simulink model "V_1_FuzzyCode"  (R2025b)
settings: Solver=VariableStepAuto  StartTime=0.0  StopTime=10.0  RelTol=1e-3
settings Model: Creator=acer  LastModifiedBy=acer

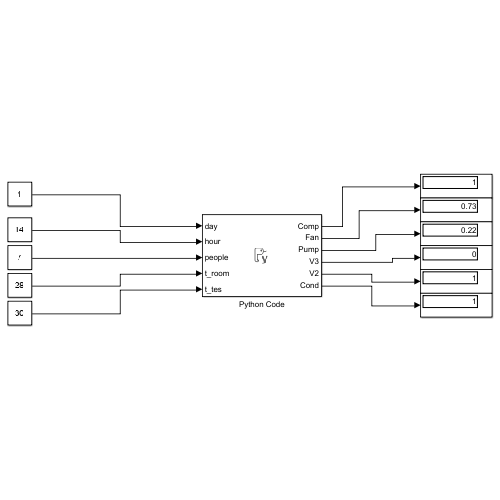
[thumbnail: Simulink's stored preview of the top-level diagram]
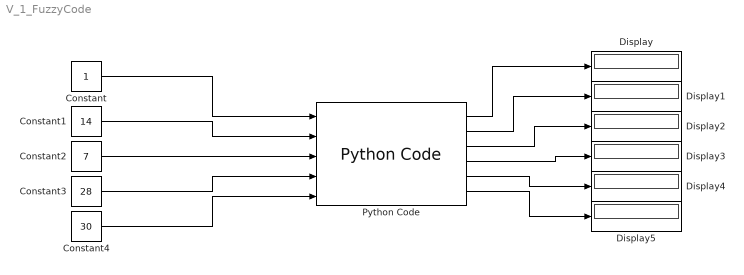
== system V_1_FuzzyCode ==
  Constant : Constant
  Constant1 : Constant  Value=14
  Constant2 : Constant  Value=7
  Constant3 : Constant  Value=28
  Constant4 : Constant  Value=30
  Display{,1..5} (6 alike) : Display
  Python Code : PythonCode  OutputCode=|
      | import numpy as np
      | import skfuzzy as fuzz
      | from skfuzzy import control as ctrl
      | 
      | # ==========================================================
      | # Persistent Fuzzy System (สร้างครั้งเดียว)
      | # ==========================================================
      | def create_fuzzy_system():
      | 
      |     # -------- INPUTS --------
      |     people = ctrl.Antecedent(np.arange(1, 32, 1), 'people')
      |     room_temp = ctrl.Antecedent(np.arange(20, 31, 1), 'room_temp')
      | 
      |     # -------- OUTPUTS --------
      |     cond_use = ctrl.Consequent(np.arange(0, 1.1, 0.1), 'cond_use')
      |     comp_use = ctrl.Consequent(np.arange(0, 1.1, 0.1), 'comp_use')
      |     pump_speed = ctrl.Consequent(np.arange(0, 101, 1), 'pump_speed')
      |     fan_speed = ctrl.Consequent(np.arange(0, 101, 1), 'fan_speed')
      |     valve_2 = ctrl.Consequent(np.arange(0, 1.1, 0.1), 'valve_2')
      |     valve_3 = ctrl.Consequent(np.arange(0, 1.1, 0.1), 'valve_3')
      | 
      |     # -------- MEMBERSHIP FUNCTIONS --------
      |     people['few'] = fuzz.trapmf(people.universe, [0, 0, 4, 6])
      |     people['medium'] = fuzz.trapmf(people.universe, [5, 10, 15, 15])
      |     people['many'] = fuzz.trapmf(people.universe, [14, 25, 31, 31])
      | 
      |     room_temp['normal'] = fuzz.trimf(room_temp.universe, [20, 20, 26])
      |     room_temp['hot'] = fuzz.trimf(room_temp.universe, [24, 27, 29])
      |     room_temp['very_hot'] = fuzz.trapmf(room_temp.universe, [28, 29, 30, 30])
      | 
      |     for output in [cond_use, comp_use, valve_2, valve_3]:
      |         output['off'] = fuzz.trimf(output.universe, [0, 0, 0.5])
      |         output['on']  = fuzz.trimf(output.universe, [0.5, 1, 1])
      | 
      |     pump_speed['low'] = fuzz.trimf(pump_speed.universe, [0, 30, 40])
      |     pump_speed['high'] = fuzz.trimf(pump_speed.universe, [30, 100, 100])
      | 
      |     fan_speed['low'] = fuzz.trimf(fan_speed.universe, [0, 30, 40])
      |     fan_speed['high'] = fuzz.trimf(fan_speed.universe, [30, 100, 100])
      | 
      |     # -------- RULES --------
      |     rules = [
      | 
      |         ctrl.Rule(people['few'] & room_temp['normal'],
      |                   [cond_use['off'], comp_use['off'], pump_speed['low'],
      |                    fan_speed['low'], valve_2['off'], valve_3['off']]),
      | 
      |         ctrl.Rule(people['medium'] & room_temp['hot'],
      |                   [cond_use['on'], comp_use['on'], pump_speed['low'],
      |                    fan_speed['high'], valve_2['on'], valve_3['off']]),
      | 
      |         ctrl.Rule(people['many'] & room_temp['very_hot'],
      |                   [cond_use['on'], comp_use['on'], pump_speed['high'],
      |                    fan_speed['high'], valve_2['on'], valve_3['off']])
      |     ]
      | 
      |     system = ctrl.ControlSystem(rules)
      |     return ctrl.ControlSystemSimulation(system)
      | 
      | 
      | # ==========================================================
      | # Controller (Time-Step Function)
      | # ==========================================================
      | fuzzy_sim = create_fuzzy_system()
      | 
      | def tes_controller(day, hour, people, t_room, t_tes):
      |     """
      |     Time-step controller (เรียกครั้งละ 1 timestep)
      | 
      |     Inputs:
      |         day     : 0-6
      |         hour    : 0-23
      |         people  : จำนวนคน
      |         t_room  : อุณหภูมิห้อง (°C)
      |         t_tes   : อุณหภูมิถัง (°C)
      | 
      |     Returns:
      |         cond, v2, v3, pump, fan, comp
      |     """
      | 
      |     # Default Output
      |     cond = 0
      |     v2 = 0
      |     v3 = 0
      |     pump = 0
      |     fan = 0
      |     comp = 0
      | 
      |     # ==============================
      |     # MODE 1 : Night Charging
      |     # ==============================
      |     if hour >= 22 or hour < 9:
      | 
      |         if people < 1:
      |             if t_tes > 5:
      |                 cond = 1
      |                 v3 = 1
      |                 comp = 1
      |         else:
      |             if t_tes > 5 and t_room > 24:
      |                 cond = 1
      |                 v2 = 1
      |                 v3 = 1
      |                 fan = 1
      |                 comp = 1
      |             elif t_tes > 5:
      |                 cond = 1
      |                 v3 = 1
      | 
      |     # ==============================
      |     # MODE 2 : Day Operation
      |     # ==============================
      |     else:
      | 
      |         if t_room > 24:
      | 
      |             fuzzy_sim.input['people'] = people
      |             fuzzy_sim.input['room_temp'] = t_room
      |             fuzzy_sim.compute()
      | 
      |             cond = int(fuzzy_sim.output['cond_use'] >= 0.5)
      |             comp = int(fuzzy_sim.output['comp_use'] >= 0.5)
      |             v2   = int(fuzzy_sim.output['valve_2'] >= 0.5)
      |             v3   = int(fuzzy_sim.output['valve_3'] >= 0.5)
      | 
      |             pump = round(fuzzy_sim.output['pump_speed'] / 100, 2)
      |             fan  = round(fuzzy_sim.output['fan_speed'] / 100, 2)
      | 
      |     return cond, v2, v3, pump, fan, comp
      | 
      | Cond,V2,V3,Pump,Fan,Comp = tes_controller(1, 14, 12, 28, 7)
  wires:
  Python Code/1 -> Display/1
  Constant/1 -> Python Code/1
  Constant1/1 -> Python Code/2
  Constant3/1 -> Python Code/4
  Constant2/1 -> Python Code/3
  Constant4/1 -> Python Code/5
  Python Code/2 -> Display1/1
  Python Code/3 -> Display2/1
  Python Code/4 -> Display3/1
  Python Code/5 -> Display4/1
  Python Code/6 -> Display5/1
